simulink model "cps_no_stereopsis_v2"  (R2012b)
settings: Solver=FixedStepDiscrete  StartTime=0.0  StopTime=8.5  FixedStep=0.1  RelTol=1e-3  SampleTimeConstraint=STIndependent
settings Model: RequirementInfo={} %GIDa_ba1ce617_85a9_495b_a3cb_2f0aceb7945f  MinMaxOverflowLogging=ForceOff  Creator=pmosterm  LastModifiedBy=pmosterm
settings SolverCC: EnableConcurrentExecution=on  ConcurrentTasks=on
settings DataIOCC: SignalLoggingSaveFormat=ModelDataLogs  SaveOutput=off  SaveTime=off
settings OptimizationCC: InlineParams=on
settings DebuggingCC: UnderspecifiedInitializationDetection=Simplified  FcnCallInpInsideContextMsg=EnableAllAsWarning  ModelReferenceExtraNoncontSigs=warning
settings ModelReferenceCC: ModelReferenceNumInstancesAllowed=Single
settings GRTTargetCC: CombineOutputUpdateFcns=off  GRTInterface=on
settings ConfigurationSet: Description=SimMechanics 2G

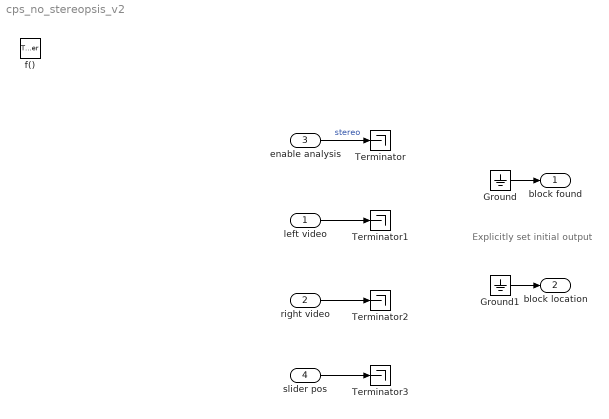
== system cps_no_stereopsis_v2 ==
  note: Explicitly set
      | initial output
  left video : Inport  OutDataTypeStr=uint8  PortDimensions=[400 240 3]
  right video : Inport  Port=2  OutDataTypeStr=uint8  PortDimensions=[400 240 3]
  enable analysis : Inport  Port=3  OutDataTypeStr=boolean  PortDimensions=1
  slider pos : Inport  Port=4  OutDataTypeStr=double  PortDimensions=1
  f() : TriggerPort  TriggerType=function-call  SampleTime=0.1  PortDimensions=1
  Ground : Ground
  Ground1 : Ground
  Terminator{,1..3} (4 alike) : Terminator
  block found : Outport  OutDataTypeStr=uint16  PortDimensions=1  InitialOutput=0
  block location : Outport  Port=2  OutDataTypeStr=double  PortDimensions=1  InitialOutput=0
  wires:
  Ground/1 -> block found/1
  Ground1/1 -> block location/1
  enable analysis/1 -> Terminator/1  "stereo"
  left video/1 -> Terminator1/1
  right video/1 -> Terminator2/1
  slider pos/1 -> Terminator3/1
